simulink model "model_microgrid"  (R2021a)
settings: Solver=FixedStepDiscrete  StartTime=1  StopTime=65705  FixedStep=1  RelTol=1e-3
settings Model: Creator=user  LastModifiedBy=user
settings DataIOCC: SignalLogging=off  DSMLogging=off  SaveTime=off  ReturnWorkspaceOutputs=off  OutputSaveName=SimulationOutput
settings SFSimCC: SimTargetLang=C++

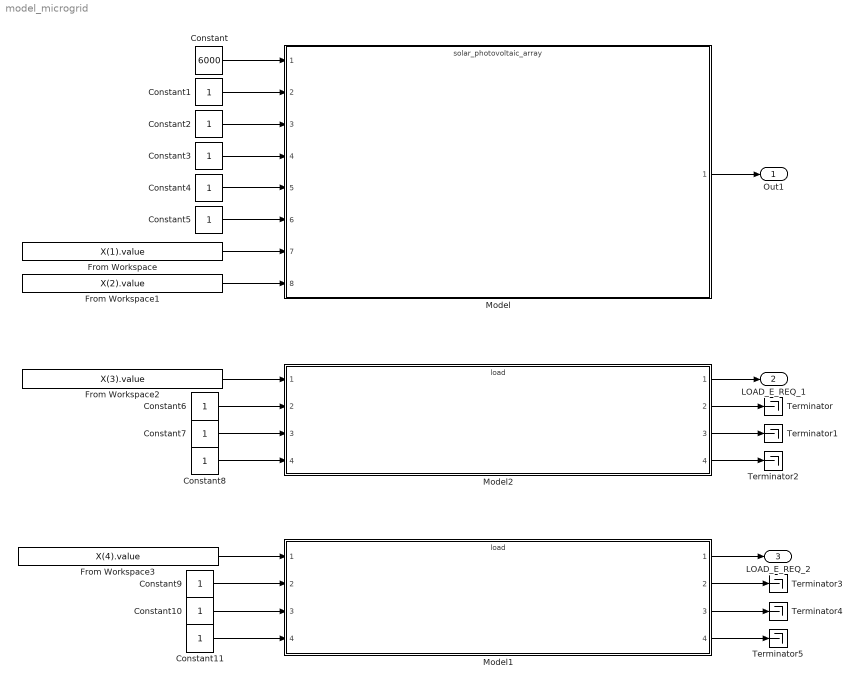
== system model_microgrid ==
  Constant : Constant  Value=6000
  Constant{1..11} (11 alike) : Constant
  From Workspace : FromWorkspace  VariableName=X(1).value  ZeroCross=off
  From Workspace1 : FromWorkspace  VariableName=X(2).value  ZeroCross=off
  From Workspace2 : FromWorkspace  VariableName=X(3).value  ZeroCross=off
  From Workspace3 : FromWorkspace  VariableName=X(4).value  ZeroCross=off
  Model : ModelReference  ModelNameDialog=solar_photovoltaic_array.slx  SimulationMode=Normal  ModelReferenceVersion=1.3
  Model1 : ModelReference  ModelNameDialog=load.slx  SimulationMode=Normal  ModelReferenceVersion=1.5
  Model2 : ModelReference  ModelNameDialog=load.slx  SimulationMode=Normal  ModelReferenceVersion=1.5
  Terminator{,1..5} (6 alike) : Terminator
  Out1 : Outport  SignalName=y1
  LOAD_E_REQ_1 : Outport  Port=2  SignalName=y2
  LOAD_E_REQ_2 : Outport  Port=3  SignalName=y3
  wires:
  Constant/1 -> Model/1
  Constant1/1 -> Model/2
  Constant2/1 -> Model/3
  Constant3/1 -> Model/4
  Constant4/1 -> Model/5
  Constant5/1 -> Model/6
  From Workspace/1 -> Model/7
  From Workspace1/1 -> Model/8
  Model/1 -> Out1/1
  From Workspace2/1 -> Model2/1
  Constant8/1 -> Model2/4
  Constant7/1 -> Model2/3
  Constant6/1 -> Model2/2
  Model2/2 -> Terminator/1
  Model2/4 -> Terminator2/1
  Model2/3 -> Terminator1/1
  Model2/1 -> LOAD_E_REQ_1/1
  Constant9/1 -> Model1/2
  Constant10/1 -> Model1/3
  From Workspace3/1 -> Model1/1
  Constant11/1 -> Model1/4
  Model1/1 -> LOAD_E_REQ_2/1
  Model1/2 -> Terminator3/1
  Model1/3 -> Terminator4/1
  Model1/4 -> Terminator5/1
